simulink model "func5_c"  (R2023a)
settings: Solver=VariableStepAuto  StartTime=0.0  StopTime=10.0  RelTol=1e-3  EnableMultiTasking=on
libraries: vmcUtilities x2, templatized_input_5_lib x1
settings Model: Creator=abehbood  LastModifiedBy=robg
settings SolverCC: AlgebraicLoopSolver=TrustRegion
settings DataIOCC: ReturnWorkspaceOutputs=off
settings OptimizationCC: LifeSpan=inf
settings DebuggingCC: UnconnectedInputMsg=warning  UnconnectedOutputMsg=warning  UnconnectedLineMsg=warning  SFUnexpectedBacktrackingDiag=warning  SFNoUnconditionalDefaultTransitionDiag=warning  ArithmeticOperatorsInVariantConditions=warning
settings ModelReferenceCC: EnableRefExpFcnMdlSchedulingChecks=on
settings SFSimCC: SimUseLocalCustomCode=off  CustomCodeUndefinedFunction=UseInterfaceOnly
settings RTWCC: RTWUseLocalCustomCode=off  DLArmComputeVersion=19.05
settings CodeAppCC: StateflowObjectComments=on
settings GRTTargetCC: TargetLangStandard=C89/C90 (ANSI)
settings ConfigComp: CovMetricSettings=dw  CovSaveCumulativeToWorkspaceVar=on  CovSaveSingleToWorkspaceVar=on  CovExternalEMLEnable=off

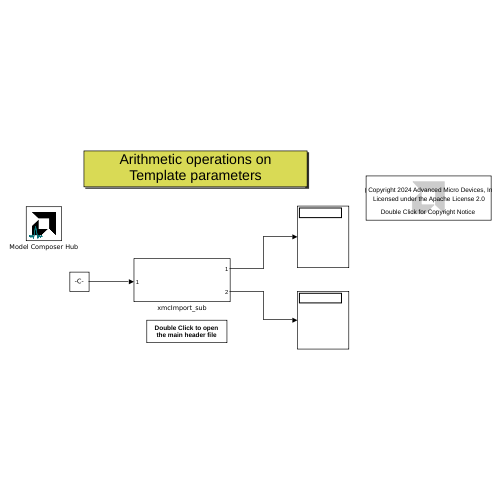
[thumbnail: Simulink's stored preview of the top-level diagram]
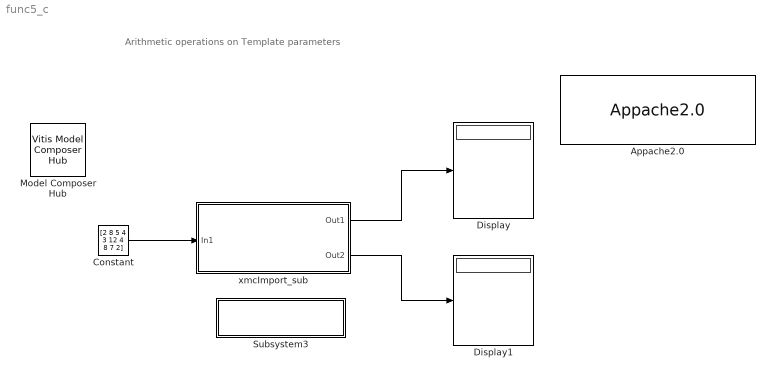
== system func5_c ==
  note: Arithmetic operations on
      | Template parameters
  Appache2.0 : vmcUtilities/Appache2.0
  Constant : Constant  Value=[2 8 5 4 3 12 4 8 7 2]  OutDataTypeStr=int16  SampleTime=1
  Display : Display
  Display1 : Display
  Model Composer Hub : vmcUtilities/Vitis Model Composer Hub  Tag=genX  CodeGeneration=off  SubsystemName=xmcImport_sub  StartColumn=1  NumberOfColumns=1  TargetDirectory=./code  exportDesign=off  analyzeDesign=off  validateDesignOnHw=off  ExportType=IP Catalog  IpVendor=xilinx.com  IpLibrary=hls  IpVersion=1.0  IpHWLanguage=Verilog  AieCompilerOptions={}  AieSimulatorOptions={}  CreateTestbench=off  TestbenchStackSize=10  RunRtlSim=off  RunCSim=off  RunAieSim=off  AieSimTimeout=50000  RunAieSimProfiling=off  LaunchVitisAnalyzer=off  PlotOutput=off  RunX86Sim=off  X86SimTimeout=10  GenHwImage=off  GenLibadfXo=off  GenHwValidationCode=off  PlatformType=Not Specified  HwSystemType=Baremetal  HwValidationTarget=hw  ProjDevice=xcku11p-ffva1156-1-e  ProjDevicePart=xcku11p-ffva1156-1-e  SamplePeriod=-1  ClockFrequency=200  DataPathParallelism=1  xilinxfamily=Kintex7  part=xc7k325t  speed=-3  package=fbg676  directory=./netlist  testbench=off  incr_netlist=off  synthesis_tool=Vivado  clock_wrapper=Clock Enables  dbl_ovrd=According to Block Masks  dcm_input_clock_period=10  sysclk_period=10  simulink_period=1  eval_field=0  LogFileName=''  NThreads=4
  Subsystem3 : Subsystem
      settings: OpenFcn=xmcOpenFileEx
      mask Display: disp(sprintf('Double Click to open\nthe main header file'))
  xmcImport_sub : Subsystem
  wires:
  Constant/1 -> xmcImport_sub/1(In1)
  xmcImport_sub/1(Out1) -> Display/1
  xmcImport_sub/2(Out2) -> Display1/1

== system func5_c/Subsystem3 ==

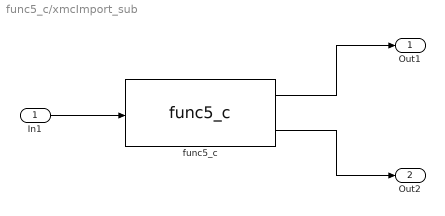
== system func5_c/xmcImport_sub ==
  In1 : Inport
  func5_c : templatized_input_5_lib/func5_c  LibraryFunction=func5_c  IncludeFiles={'func5_c.h'}  SourceFiles={}  IncludeDirectories={}  TemplateParams={'int NUMOFELEMENTS'}  FunctionParamTypes={xmcDataType('void'); xmcDataType('int16_t'); xmcDataType('int16_t'); xmcDataType('int16_t')}  FunctionParamPassbys={0.000000000000000000e+00; 0.000000000000000000e+00; 0.000000000000000000e+00; 0.000000000000000000e+00}  FunctionParamDimensions={'1'; '[NUMOFELEMENTS]'; '[NUMOFELEMENTS / 2]'; '[2 * NUMOFELEMENTS - 15]'}  FunctionParamNames={'return'; 'in'; 'out0'; 'out1'}  FunctionParamDir={0.000000000000000000e+00; 1.000000000000000000e+00; 2.000000000000000000e+00; 2.000000000000000000e+00}  FunctionParamSupportsStreaming={false; false; false; false}  BufferDepth={'0'}  FunctionParamValues={'0'; '0'; '0'; '0'}  ThroughputFactors={''}
  Out1 : Outport
  Out2 : Outport  Port=2
  wires:
  func5_c/2 -> Out2/1
  In1/1 -> func5_c/1
  func5_c/1 -> Out1/1
